simulink model "SOFC_5kW"  (Simulink 6.2)
settings: Solver=ode23tb  StartTime=0.0  StopTime=15800  MaxStep=1  RelTol=1e-3
libraries: simulink x1
settings Model: LastModifiedBy=cwang
settings DataIOCC: SaveFinalState=on  SaveOutput=off  SaveTime=off  SignalLoggingName=sigsOut
settings HardwareCC: TargetUnknown=on

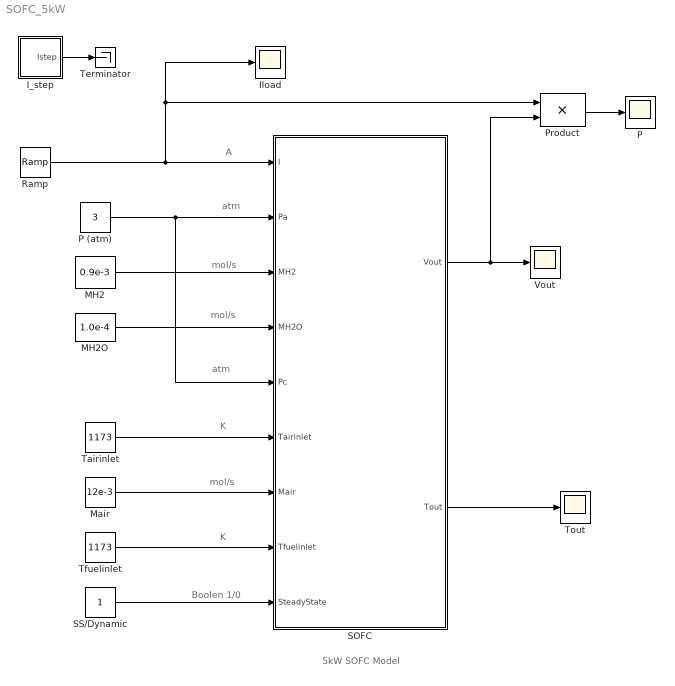
== system SOFC_5kW ==
  note: atm
  note: mol/s
  note: atm
  note: A
  note: mol/s
  note: mol/s
  note: K
  note: K
  note: 5kW SOFC Model
  note: Boolen 1/0
  I_step : Subsystem
  Iload : Scope
      settings: YMin=95  YMax=105  SaveName=Iload  DataFormat=Array
  MH2 : Constant  Value=0.9e-3
  MH2O : Constant  Value=1.0e-4
  Mair : Constant  Value=12e-3
  P : Scope
      settings: TimeRange=16000  YMin=0  YMax=5000  SaveName=Psofc  DataFormat=Array
  P (atm) : Constant  Value=3
  Product : Product  SaturateOnIntegerOverflow=on
  Ramp : simulink/Sources/Ramp  slope=0.01  start=0  X0=0
  SOFC : Subsystem
  SS/Dynamic : Constant
  Tairinlet : Constant  Value=1173
  Terminator : Terminator
  Tfuelinlet : Constant  Value=1173
  Tout : Scope
      settings: SaveName=Tout  DataFormat=Array
  Vout : Scope
      settings: SaveName=Vout  DataFormat=Array
  wires:
  P (atm)/1 -> SOFC/5(Pc), SOFC/2(Pa)
  MH2/1 -> SOFC/3(MH2)
  MH2O/1 -> SOFC/4(MH2O)
  SOFC/1(Vout) -> Vout/1, Product/2
  SOFC/2(Tout) -> Tout/1
  Tairinlet/1 -> SOFC/6(Tairinlet)
  Mair/1 -> SOFC/7(Mair)
  Tfuelinlet/1 -> SOFC/8(Tfuelinlet)
  Product/1 -> P/1
  Ramp/1 -> Iload/1, Product/1, SOFC/1(I)
  SS/Dynamic/1 -> SOFC/9(SteadyState)
  I_step/1(Istep) -> Terminator/1

== system SOFC_5kW/I_step ==
  Step : Step  Time=1000  After=80  SampleTime=0
  Step1 : Step  Time=8000  After=-50  SampleTime=0
  Sum2 : Sum  Inputs=++|  SaturateOnIntegerOverflow=on
  Istep : Outport
  wires:
  Step/1 -> Sum2/2
  Step1/1 -> Sum2/1
  Sum2/1 -> Istep/1

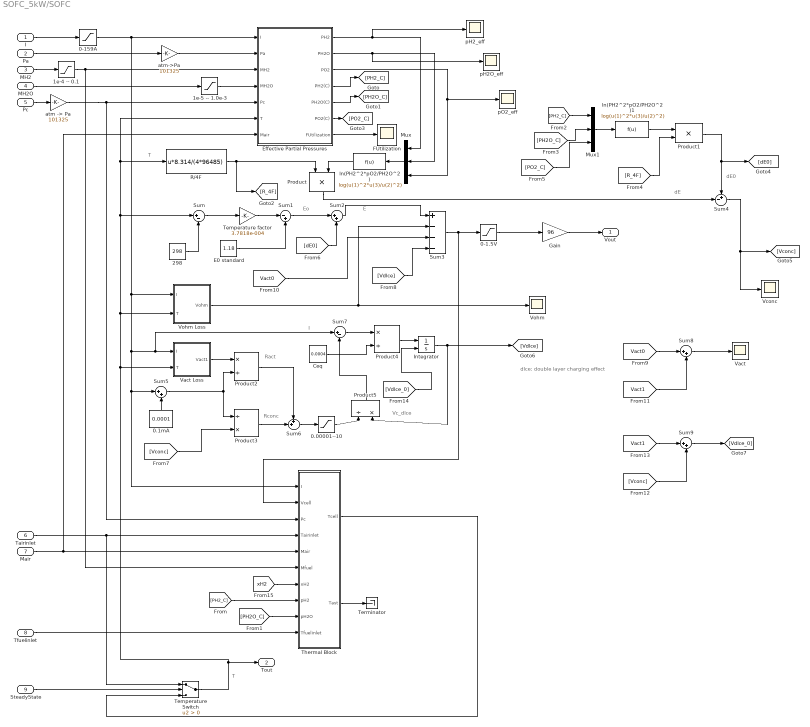
== system SOFC_5kW/SOFC ==
  note: Eo
  note: E
  note: T
  note: T
  note: dE0
  note: dE
  note: Ract
  note: Rconc
  note: I
  note: Vc_dlce
  note: dlce: double layer charging effect
  I : Inport  Port=1  LatchInput=off
  Pa : Inport  Port=2  LatchInput=off
  MH2 : Inport  Port=3  LatchInput=off
  MH2O : Inport  Port=4  LatchInput=off
  Pc : Inport  Port=5  LatchInput=off
  Tairinlet : Inport  Port=6  LatchInput=off
  Mair : Inport  Port=7  LatchInput=off
  Tfuelinlet : Inport  Port=8  LatchInput=off
  SteadyState : Inport  Port=9  LatchInput=off
  0-1.5V : Saturate  UpperLimit=1.5  LowerLimit=0
  0-159A : Saturate  UpperLimit=199  LowerLimit=0
  0.00001--10 : Saturate  UpperLimit=10  LowerLimit=0.00001
  0.1mA : Constant  Orientation=up  Value=0.0001
  "1e-4 -- 0.1" : Saturate  UpperLimit=0.1  LowerLimit=1.0e-4
  "1e-5 -- 1.0e-3" : Saturate  UpperLimit=1.0e-3  LowerLimit=1.0e-5
  298 : Constant  Value=298
  Ceq : Constant  Value=0.0004
  E0 standard : Constant  Value=1.18
  Effective Partial Pressures : Subsystem
  FUtilization : Scope
      settings: SaveName=FUtilization
  Gain : Gain  Gain=96  SaturateOnIntegerOverflow=on
  Integrator : Integrator  InitialConditionSource=external
  Mux : Mux  Orientation=left  Inputs=3
  Mux1 : Mux  Inputs=3
  Product : Product  Orientation=down  SaturateOnIntegerOverflow=on
  Product1 : Product  SaturateOnIntegerOverflow=on
  Product2 : Product  Inputs=*/  SaturateOnIntegerOverflow=on
  Product3 : Product  Inputs=/*  SaturateOnIntegerOverflow=on
  Product4 : Product  Inputs=*/  SaturateOnIntegerOverflow=on
  Product5 : Product  Orientation=up  Inputs=/*  SaturateOnIntegerOverflow=on
  R/4F : Fcn  Expr=u*8.314/(4*96485)
  Sum : Sum  Inputs=|+-  SaturateOnIntegerOverflow=on
  Sum1 : Sum  Inputs=|-+  SaturateOnIntegerOverflow=on
  Sum{2,5,8..9} (4 alike) : Sum  Inputs=|++  SaturateOnIntegerOverflow=on
  Sum3 : Sum  Inputs=+---  SaturateOnIntegerOverflow=on
  Sum4 : Sum  Inputs=+-|  SaturateOnIntegerOverflow=on
  Sum6 : Sum  Inputs=++|  SaturateOnIntegerOverflow=on
  Sum7 : Sum  Inputs=|+-  SaturateOnIntegerOverflow=on
  Temperature Switch : Switch  Criteria=u2 > Threshold  SaturateOnIntegerOverflow=on
  Temperature factor : Gain  Gain=3.7818e-004  SaturateOnIntegerOverflow=on
  Terminator : Terminator
  Thermal Block : Subsystem
  Vact : Scope
      settings: YMin=0  YMax=0.6  SaveName=Vact  DataFormat=Array
  Vact Loss : Subsystem
  Vconc : Scope
      settings: YMin=0  YMax=0.6  SaveName=Vconc  DataFormat=Array
  Vohm : Scope
      settings: YMin=0  YMax=0.6  SaveName=Vohm  DataFormat=Array
  Vohm Loss : Subsystem
  "atm -> Pa" : Gain  Gain=101325  SaturateOnIntegerOverflow=on
  atm->Pa : Gain  Gain=101325  SaturateOnIntegerOverflow=on
  ln(PH2^2*pO2/PH2O^2) : Fcn  Orientation=left  Expr=log(u(1)^2*u(3)/u(2)^2)
  ln(PH2^2*pO2/PH2O^2)1 : Fcn  Expr=log(u(1)^2*u(3)/u(2)^2)
  pH2O_eff : Scope
      settings: SaveName=pH2O_eff
  pH2_eff : Scope
      settings: TimeRange=9.779411764705881  YMin=75033  YMax=75199.9  SaveName=pH2_eff  DataFormat=Array  MaxDataPoints=10000
  pO2_eff : Scope
      settings: SaveName=pO2_eff
  Vout : Outport
  Tout : Outport  Port=2
  wires:
  Effective Partial Pressures/1(PH2) -> Mux/1, pH2_eff/1
  Pa/1 -> atm->Pa/1
  MH2/1 -> "1e-4 -- 0.1"/1
  MH2O/1 -> "1e-5 -- 1.0e-3"/1
  Effective Partial Pressures/2(PH2O) -> Mux/2, pH2O_eff/1
  Pc/1 -> "atm -> Pa"/1
  Effective Partial Pressures/3(PO2) -> pO2_eff/1, Mux/3
  298/1 -> Sum/2
  Sum/1 -> Temperature factor/1
  Temperature factor/1 -> Sum1/1
  E0 standard/1 -> Sum1/2
  Mux/1 -> ln(PH2^2*pO2/PH2O^2)/1
  R/4F/1 -> Product/1, [R_4F]
  ln(PH2^2*pO2/PH2O^2)/1 -> Product/2
  Product/1 -> Sum4/2
  I/1 -> 0-159A/1
  Sum2/1 -> Sum3/1
  Vohm Loss/1(Vohm) -> Sum3/2, Vohm/1
  Sum3/1 -> Thermal Block/2(Vcell), 0-1.5V/1
  Thermal Block/2(Tast) -> Terminator/1
  Thermal Block/1(Tcell) -> Temperature Switch/3
  atm->Pa/1 -> Effective Partial Pressures/2(Pa)
  Tairinlet/1 -> Thermal Block/4(Tairinlet), Temperature Switch/1
  Mair/1 -> Thermal Block/5(Mair), Effective Partial Pressures/7(Mair)
  "atm -> Pa"/1 -> Thermal Block/3(Pc), Effective Partial Pressures/5(Pc)
  Tfuelinlet/1 -> Thermal Block/10(Tfuelinlet)
  Effective Partial Pressures/4(PH2(C)) -> [PH2_C]
  Effective Partial Pressures/5(PH2O(C)) -> [PH2O_C]
  [PH2_C] -> Thermal Block/8(pH2)
  [PH2O_C] -> Thermal Block/9(pH2O)
  0-159A/1 -> Thermal Block/1(I), Sum5/1, Vact Loss/1(I), Sum7/1, Vohm Loss/1(I), Effective Partial Pressures/1(I)
  0-1.5V/1 -> Gain/1
  SteadyState/1 -> Temperature Switch/2
  Temperature Switch/1 -> Vohm Loss/2(T), Sum/1, Effective Partial Pressures/6(T), R/4F/1, Vact Loss/2(T), Tout/1
  Effective Partial Pressures/6(PO2(C)) -> [PO2_C]
  [PH2_C] -> Mux1/1
  [PH2O_C] -> Mux1/2
  Mux1/1 -> ln(PH2^2*pO2/PH2O^2)1/1
  ln(PH2^2*pO2/PH2O^2)1/1 -> Product1/1
  [R_4F] -> Product1/2
  Product1/1 -> Sum4/1, [dE0]
  Sum4/1 -> [Vconc], Vconc/1
  [PO2_C] -> Mux1/3
  "1e-5 -- 1.0e-3"/1 -> Effective Partial Pressures/4(MH2O)
  Effective Partial Pressures/7(FUtilization) -> FUtilization/1
  Sum1/1 -> Sum2/1
  [dE0] -> Sum2/2
  Vact Loss/1(Vact1) -> Product2/1
  0.1mA/1 -> Sum5/2
  Sum5/1 -> Product2/2, Product3/1
  Product2/1 -> Sum6/1
  [Vconc] -> Product3/2
  Sum7/1 -> Product4/1
  Ceq/1 -> Product4/2
  Product4/1 -> Integrator/1
  [Vdlce_0] -> Integrator/2
  Product3/1 -> Sum6/2
  Sum6/1 -> 0.00001--10/1
  0.00001--10/1 -> Product5/1
  Integrator/1 -> Product5/2, [Vdlce]
  Product5/1 -> Sum7/2
  [Vact0] -> Sum3/3
  [Vdlce] -> Sum3/4
  [Vact0] -> Sum8/1
  [Vact1] -> Sum8/2
  Sum8/1 -> Vact/1
  [Vact1] -> Sum9/1
  [Vconc] -> Sum9/2
  Sum9/1 -> [Vdlce_0]
  "1e-4 -- 0.1"/1 -> Effective Partial Pressures/3(MH2), Thermal Block/6(Mfuel)
  [xH2] -> Thermal Block/7(xH2)
  Gain/1 -> Vout/1

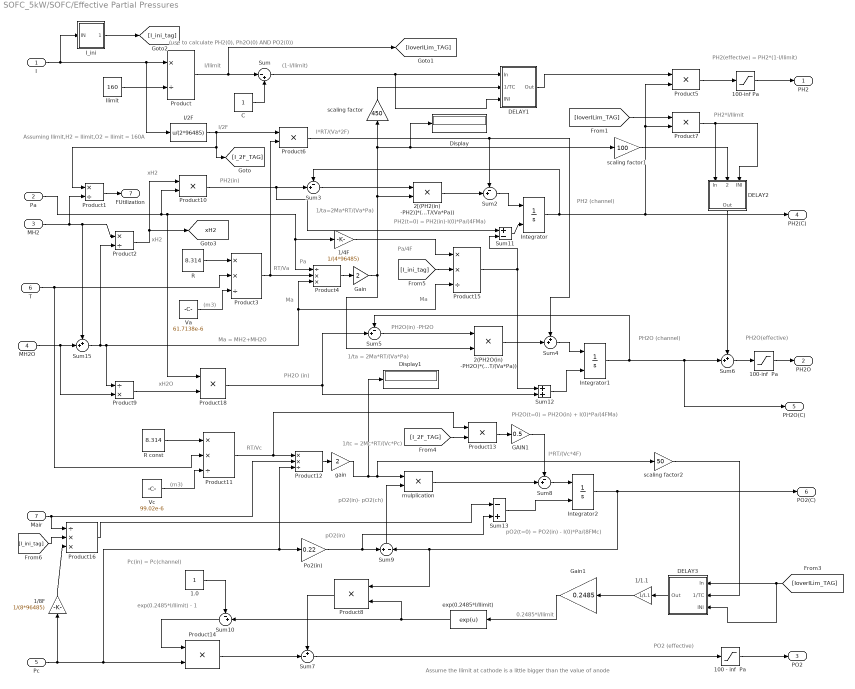
== system SOFC_5kW/SOFC/Effective Partial Pressures ==
  note: RT/Va
  note: PH2(in)
  note: 1/ta = 2Ma*RT/(Va*Pa)
  note: Pa
  note: Ma
  note: PH2(t=0) = PH2(in)-I(0)*Pa/(4FMa)
  note: I/2F
  note: I*RT/(Va*2F)
  note: PH2 (channel)
  note: PH2O(in) -PH2O
  note: PH2O(t=0) = PH2O(in) + I(0)*Pa/(4FMa)
  note: PH2O (channel)
  note: (1-I/Ilimit)
  note: Assuming Ilimit,H2 = Ilimit,O2
      |       = Ilimit = 160A
  note: I/Ilimit
  note: PH2*I/Ilimit
  note: PH2(effective) = PH2*(1-I/Ilimit)
  note: PH2O(effective)
  note: Ma = MH2+MH2O
  note: Pc(in) = Pc(channel)
  note: Assume the Ilimit at cathode is a little bigger than the value of anode
  note: 0.2485*I/Ilimit
  note: PO2 (effective)
  note: (m3)
  note: RT/Vc
  note: (m3)
  note: pO2(in)- pO2(ch)
  note: 1/tc = 2Mc*RT/(Vc*Pc)
  note: I*RT/(Vc*4F)
  note: exp(0.2485*I/Ilimit) - 1
  note: (use to calculate PH2(0), Ph2O(0) AND PO2(0))
  note: Pa/4F
  note: Ma
  note: PH2O (in)
  note: pO2(in)
  note: pO2(t=0) = PO2(in) - I(0)*Pa/(8FMc)
  note: 1/ta=2Ma*RT/(Va*Pa)
  note: xH2
  note: xH2
  note: xH2O
  I : Inport  Port=1  LatchInput=off
  Pa : Inport  Port=2  LatchInput=off
  MH2 : Inport  Port=3  LatchInput=off
  MH2O : Inport  Port=4  LatchInput=off
  Pc : Inport  Port=5  LatchInput=off
  T : Inport  Port=6  LatchInput=off
  Mair : Inport  Port=7  LatchInput=off
  1.0 : Constant
  1/1.1 : Gain  Orientation=left  Gain=1/1.1  SaturateOnIntegerOverflow=on
  1/4F : Gain  Gain=1/(4*96485)  SaturateOnIntegerOverflow=on
  1/8F : Gain  Orientation=up  Gain=1/(8*96485)  SaturateOnIntegerOverflow=on
  100 - inf  Pa : Saturate  UpperLimit=inf  LowerLimit=100
  100-inf  Pa : Saturate  UpperLimit=inf  LowerLimit=100
  100-inf Pa : Saturate  UpperLimit=inf  LowerLimit=100
  2(PH2O(in) -PH2O)*(Ma*RT/(Va*Pa)) : Product  SaturateOnIntegerOverflow=on
  2[(PH2(in) -PH2)]*(Ma*RT/(Va*Pa)) : Product  SaturateOnIntegerOverflow=on
  C : Constant
  DELAY1 : Subsystem
  DELAY2 : Subsystem  Orientation=down
  DELAY3 : Subsystem  Orientation=left
  Display : Display
  Display1 : Display
  GAIN1 : Gain  Gain=0.5  SaturateOnIntegerOverflow=on
  Gain : Gain  Gain=2  SaturateOnIntegerOverflow=on
  Gain1 : Gain  Orientation=left  Gain=0.2485  SaturateOnIntegerOverflow=on
  I/2F : Fcn  Expr=u/(2*96485)
  I_ini : Subsystem
  Ilimit : Constant  Value=160
  Integrator : Integrator  InitialConditionSource=external
  Integrator1 : Integrator  InitialConditionSource=external
  Integrator2 : Integrator  InitialConditionSource=external
  Po2(in) : Gain  Gain=0.22  SaturateOnIntegerOverflow=on
  Product : Product  Inputs=*/  SaturateOnIntegerOverflow=on
  Product1 : Product  Inputs=*/  SaturateOnIntegerOverflow=on
  Product{5..7,10,13..14,18} (7 alike) : Product  SaturateOnIntegerOverflow=on
  Product{3,11..12,15} (4 alike) : Product  Inputs=**/  SaturateOnIntegerOverflow=on
  Product16 : Product  Inputs=/**  SaturateOnIntegerOverflow=on
  Product2 : Product  Inputs=*/  SaturateOnIntegerOverflow=on
  Product4 : Product  Inputs=/**  SaturateOnIntegerOverflow=on
  Product8 : Product  Orientation=left  SaturateOnIntegerOverflow=on
  Product9 : Product  Inputs=/*  SaturateOnIntegerOverflow=on
  R : Constant  Value=8.314
  R const : Constant  Value=8.314
  Sum : Sum  Inputs=|-+  SaturateOnIntegerOverflow=on
  Sum10 : Sum  Orientation=left  Inputs=-+|  SaturateOnIntegerOverflow=on
  Sum11 : Sum  Inputs=+-  SaturateOnIntegerOverflow=on
  Sum12 : Sum  SaturateOnIntegerOverflow=on
  Sum13 : Sum  Inputs=-+  SaturateOnIntegerOverflow=on
  Sum15 : Sum  Inputs=++|  SaturateOnIntegerOverflow=on
  Sum{2..3,5,8} (4 alike) : Sum  Inputs=-+|  SaturateOnIntegerOverflow=on
  Sum4 : Sum  Inputs=++|  SaturateOnIntegerOverflow=on
  Sum6 : Sum  Inputs=++|  SaturateOnIntegerOverflow=on
  Sum7 : Sum  Inputs=+-|  SaturateOnIntegerOverflow=on
  Sum9 : Sum  Orientation=up  Inputs=+|-  SaturateOnIntegerOverflow=on
  Va : Constant  Value=61.7138e-6
  Vc : Constant  Value=99.02e-6
  exp(0.2485*I/Ilimit) : Fcn  Orientation=left  Expr=exp(u)
  gain : Gain  Gain=2  SaturateOnIntegerOverflow=on
  mulplication : Product  SaturateOnIntegerOverflow=on
  scaling factor : Gain  Orientation=up  Gain=450  SaturateOnIntegerOverflow=on
  scaling factor1 : Gain  Gain=100  SaturateOnIntegerOverflow=on
  scaling factor2 : Gain  Gain=50  SaturateOnIntegerOverflow=on
  PH2 : Outport
  PH2O : Outport  Port=2
  PO2 : Outport  Port=3
  PH2(C) : Outport  Port=4
  PH2O(C) : Outport  Port=5
  PO2(C) : Outport  Port=6
  FUtilization : Outport  Port=7
  tag scope: xH2=global
  wires:
  I/1 -> Product/1, I/2F/1, I_ini/1(IN)
  Ilimit/1 -> Product/2
  Product/1 -> Sum/1, [IoverILim_TAG]
  C/1 -> Sum/2
  R/1 -> Product3/1
  T/1 -> Product3/2, Product11/2
  Va/1 -> Product3/3
  Product4/1 -> Gain/1
  Product3/1 -> Product4/2, Product6/2
  Product10/1 -> Sum11/1, Sum3/2
  Sum3/1 -> 2[(PH2(in) -PH2)]*(Ma*RT/(Va*Pa))/1
  2[(PH2(in) -PH2)]*(Ma*RT/(Va*Pa))/1 -> Sum2/2
  I/2F/1 -> Product6/1, [I_2F_TAG], Product1/1
  Product6/1 -> Sum2/1, Sum4/1
  Integrator/1 -> Sum3/1, Product5/2, Product7/2, PH2(C)/1
  Sum2/1 -> Integrator/1
  Product18/1 -> Sum5/2, Sum12/2
  Sum5/1 -> 2(PH2O(in) -PH2O)*(Ma*RT/(Va*Pa))/1
  2(PH2O(in) -PH2O)*(Ma*RT/(Va*Pa))/1 -> Sum4/2
  Integrator1/1 -> Sum5/1, Sum6/2, PH2O(C)/1
  Sum4/1 -> Integrator1/1
  Product5/1 -> 100-inf Pa/1
  Sum6/1 -> 100-inf  Pa/1
  Pc/1 -> Product14/2, Product12/3, Po2(in)/1, 1/8F/1
  Gain1/1 -> exp(0.2485*I/Ilimit)/1
  Sum7/1 -> 100 - inf  Pa/1
  100-inf Pa/1 -> PH2/1
  100-inf  Pa/1 -> PH2O/1
  100 - inf  Pa/1 -> PO2/1
  [IoverILim_TAG] -> Product7/1
  R const/1 -> Product11/1
  Vc/1 -> Product11/3
  Product11/1 -> Product12/1, Product13/1
  Mair/1 -> Product12/2, Product16/1
  Product12/1 -> gain/1
  gain/1 -> mulplication/1, scaling factor2/1, Display1/1
  Integrator2/1 -> PO2(C)/1, Sum9/2, Product8/1
  Po2(in)/1 -> Sum9/1, Sum13/2
  Sum9/1 -> mulplication/2
  mulplication/1 -> Sum8/2
  [I_2F_TAG] -> Product13/2
  Product13/1 -> GAIN1/1
  GAIN1/1 -> Sum8/1
  Sum8/1 -> Integrator2/1
  exp(0.2485*I/Ilimit)/1 -> Sum10/2, Product8/2
  Sum10/1 -> Product14/1
  1.0/1 -> Sum10/1
  Product14/1 -> Sum7/2
  Product8/1 -> Sum7/1
  I_ini/1(IN(0)) -> [I_ini_tag]
  Sum11/1 -> Integrator/2
  1/4F/1 -> Product15/1
  [I_ini_tag] -> Product15/2
  Product15/1 -> Sum11/2, Sum12/1
  Sum12/1 -> Integrator1/2
  [I_ini_tag] -> Product16/2
  1/8F/1 -> Product16/3
  Product16/1 -> Sum13/1
  Sum13/1 -> Integrator2/2
  1/1.1/1 -> Gain1/1
  Gain/1 -> 2(PH2O(in) -PH2O)*(Ma*RT/(Va*Pa))/2, 2[(PH2(in) -PH2)]*(Ma*RT/(Va*Pa))/2, scaling factor/1, scaling factor1/1, Display/1
  Sum/1 -> DELAY1/1(In), DELAY1/3(INI)
  DELAY1/1(Out) -> Product5/1
  Product7/1 -> DELAY2/1(In), DELAY2/3(INI)
  DELAY2/1(Out) -> Sum6/1
  [IoverILim_TAG] -> DELAY3/1(In), DELAY3/3(INI)
  DELAY3/1(Out) -> 1/1.1/1
  scaling factor/1 -> DELAY1/2(1/TC)
  scaling factor1/1 -> DELAY2/2(1/TC)
  scaling factor2/1 -> DELAY3/2(1/TC)
  Sum15/1 -> Product2/2, Product4/3, Product15/3, Product9/1
  MH2O/1 -> Sum15/2, Product9/2
  MH2/1 -> Sum15/1, Product2/1, Product1/2
  Product2/1 -> Product10/1, [xH2]
  Pa/1 -> Product10/2, Product4/1, 1/4F/1, Product18/1
  Product9/1 -> Product18/2
  Product1/1 -> FUtilization/1

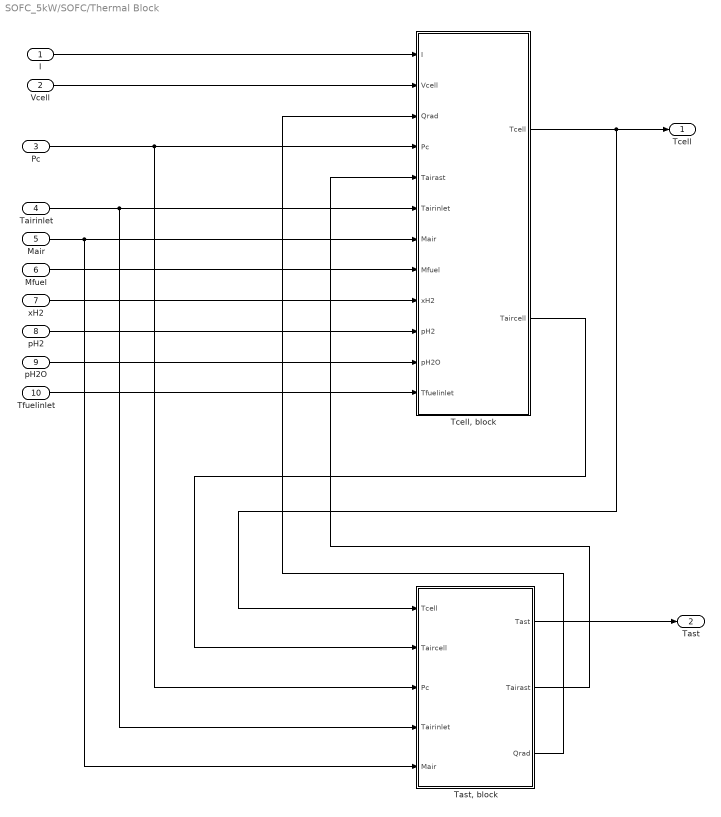
== system SOFC_5kW/SOFC/Thermal Block ==
  I : Inport  Port=1  LatchInput=off
  Vcell : Inport  Port=2  LatchInput=off
  Pc : Inport  Port=3  LatchInput=off
  Tairinlet : Inport  Port=4  LatchInput=off
  Mair : Inport  Port=5  LatchInput=off
  Mfuel : Inport  Port=6  LatchInput=off
  xH2 : Inport  Port=7  LatchInput=off
  pH2 : Inport  Port=8  LatchInput=off
  pH2O : Inport  Port=9  LatchInput=off
  Tfuelinlet : Inport  Port=10  LatchInput=off
  "Tast, block" : Subsystem
  "Tcell, block" : Subsystem
  Tcell : Outport
  Tast : Outport  Port=2
  wires:
  "Tast, block"/1(Tast) -> Tast/1
  I/1 -> "Tcell, block"/1(I)
  Vcell/1 -> "Tcell, block"/2(Vcell)
  "Tast, block"/2(Tairast) -> "Tcell, block"/5(Tairast)
  "Tast, block"/3(Qrad) -> "Tcell, block"/3(Qrad)
  "Tcell, block"/1(Tcell) -> "Tast, block"/1(Tcell), Tcell/1
  "Tcell, block"/2(Taircell) -> "Tast, block"/2(Taircell)
  Pc/1 -> "Tcell, block"/4(Pc), "Tast, block"/3(Pc)
  Tairinlet/1 -> "Tcell, block"/6(Tairinlet), "Tast, block"/4(Tairinlet)
  Mair/1 -> "Tcell, block"/7(Mair), "Tast, block"/5(Mair)
  Mfuel/1 -> "Tcell, block"/8(Mfuel)
  xH2/1 -> "Tcell, block"/9(xH2)
  pH2/1 -> "Tcell, block"/10(pH2)
  pH2O/1 -> "Tcell, block"/11(pH2O)
  Tfuelinlet/1 -> "Tcell, block"/12(Tfuelinlet)

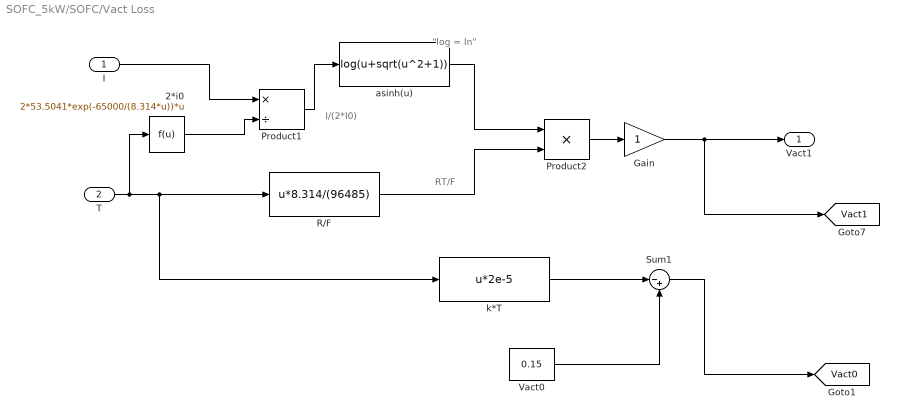
== system SOFC_5kW/SOFC/Vact Loss ==
  note: RT/F
  note: "log = ln"
  note: I/(2*I0)
  I : Inport  Port=1  LatchInput=off
  T : Inport  Port=2  LatchInput=off
  2*i0 : Fcn  Expr=2*53.5041*exp(-65000/(8.314*u))*u
  Gain : Gain  SaturateOnIntegerOverflow=on
  Product1 : Product  Inputs=*/  SaturateOnIntegerOverflow=on
  Product2 : Product  SaturateOnIntegerOverflow=on
  R/F : Fcn  Expr=u*8.314/(96485)
  Sum1 : Sum  Inputs=|-+  SaturateOnIntegerOverflow=on
  Vact0 : Constant  Value=0.15
  asinh(u) : Fcn  Expr=log(u+sqrt(u^2+1))
  k*T : Fcn  Expr=u*2e-5
  Vact1 : Outport
  tag scope: Vact0=global, Vact1=global
  wires:
  T/1 -> k*T/1, R/F/1, 2*i0/1
  R/F/1 -> Product2/2
  I/1 -> Product1/1
  Product2/1 -> Gain/1
  asinh(u)/1 -> Product2/1
  Product1/1 -> asinh(u)/1
  Gain/1 -> Vact1/1, [Vact1]
  k*T/1 -> Sum1/1
  Vact0/1 -> Sum1/2
  Sum1/1 -> [Vact0]
  2*i0/1 -> Product1/2

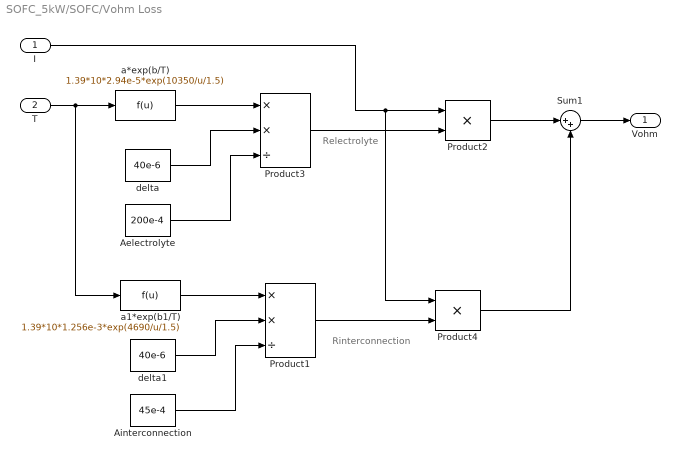
== system SOFC_5kW/SOFC/Vohm Loss ==
  note: Relectrolyte
  note: Rinterconnection
  I : Inport  Port=1  LatchInput=off
  T : Inport  Port=2  LatchInput=off
  Aelectrolyte : Constant  Value=200e-4
  Ainterconnection : Constant  Value=45e-4
  Product1 : Product  Inputs=**/  SaturateOnIntegerOverflow=on
  Product2 : Product  SaturateOnIntegerOverflow=on
  Product3 : Product  Inputs=**/  SaturateOnIntegerOverflow=on
  Product4 : Product  SaturateOnIntegerOverflow=on
  Sum1 : Sum  Inputs=|++  SaturateOnIntegerOverflow=on
  a*exp(b/T) : Fcn  Expr=1.39*10*2.94e-5*exp(10350/u/1.5)
  a1*exp(b1/T) : Fcn  Expr=1.39*10*1.256e-3*exp(4690/u/1.5)
  delta : Constant  Value=40e-6
  delta1 : Constant  Value=40e-6
  Vohm : Outport
  wires:
  T/1 -> a1*exp(b1/T)/1, a*exp(b/T)/1
  a*exp(b/T)/1 -> Product3/1
  delta/1 -> Product3/2
  Aelectrolyte/1 -> Product3/3
  Product3/1 -> Product2/2
  a1*exp(b1/T)/1 -> Product1/1
  delta1/1 -> Product1/2
  Ainterconnection/1 -> Product1/3
  Product1/1 -> Product4/2
  I/1 -> Product4/1, Product2/1
  Product2/1 -> Sum1/1
  Product4/1 -> Sum1/2
  Sum1/1 -> Vohm/1

== system SOFC_5kW/SOFC/Effective Partial Pressures/DELAY1 ==
  note: time constant
  In : Inport  Port=1  LatchInput=off
  1/TC : Inport  Port=2  LatchInput=off
  INI : Inport  Port=3  LatchInput=off
  Integrator : Integrator  InitialConditionSource=external
  Product1 : Product  SaturateOnIntegerOverflow=on
  Sum : Sum  Inputs=|+-  SaturateOnIntegerOverflow=on
  Out : Outport
  wires:
  Sum/1 -> Product1/2
  Integrator/1 -> Sum/2, Out/1
  Product1/1 -> Integrator/1
  1/TC/1 -> Product1/1
  In/1 -> Sum/1
  INI/1 -> Integrator/2

== system SOFC_5kW/SOFC/Effective Partial Pressures/DELAY2 ==
  note: time constant
  In : Inport  Port=1  LatchInput=off
  1/TC : Inport  Port=2  LatchInput=off
  INI : Inport  Port=3  LatchInput=off
  Integrator : Integrator  InitialConditionSource=external
  Product1 : Product  SaturateOnIntegerOverflow=on
  Sum : Sum  Inputs=|+-  SaturateOnIntegerOverflow=on
  Out : Outport
  wires:
  Sum/1 -> Product1/2
  Integrator/1 -> Sum/2, Out/1
  Product1/1 -> Integrator/1
  1/TC/1 -> Product1/1
  In/1 -> Sum/1
  INI/1 -> Integrator/2

== system SOFC_5kW/SOFC/Effective Partial Pressures/DELAY3 ==
  note: time constant
  In : Inport  Port=1  LatchInput=off
  1/TC : Inport  Port=2  LatchInput=off
  INI : Inport  Port=3  LatchInput=off
  Integrator : Integrator  InitialConditionSource=external
  Product1 : Product  SaturateOnIntegerOverflow=on
  Sum : Sum  Inputs=|+-  SaturateOnIntegerOverflow=on
  Out : Outport
  wires:
  Sum/1 -> Product1/2
  Integrator/1 -> Sum/2, Out/1
  Product1/1 -> Integrator/1
  1/TC/1 -> Product1/1
  In/1 -> Sum/1
  INI/1 -> Integrator/2

== system SOFC_5kW/SOFC/Effective Partial Pressures/I_ini ==
  IN : Inport  Port=1  LatchInput=off
  Integrator : Integrator  InitialConditionSource=external
  zero : Constant  Value=0
  IN(0) : Outport
  wires:
  zero/1 -> Integrator/1
  Integrator/1 -> IN(0)/1
  IN/1 -> Integrator/2

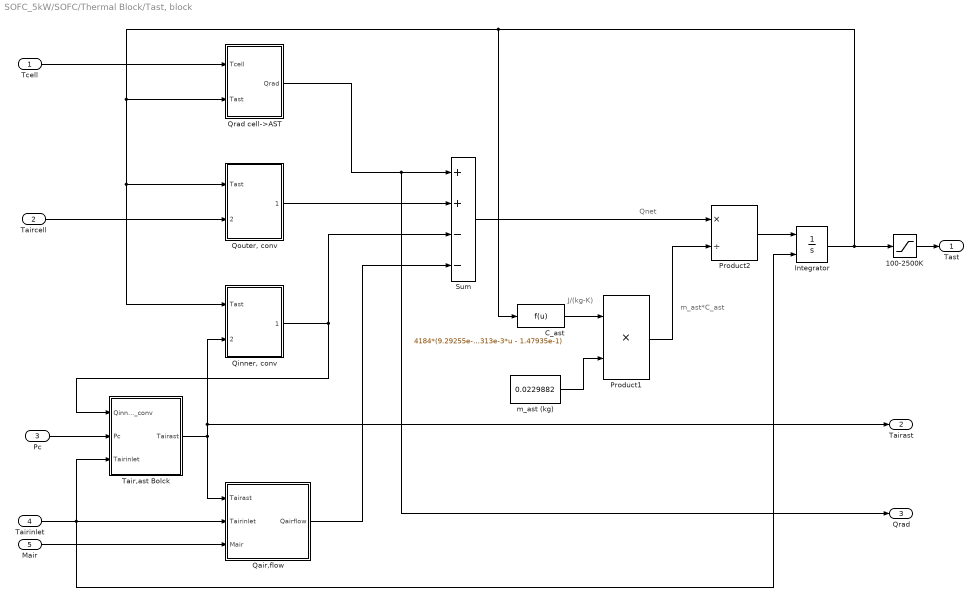
== system SOFC_5kW/SOFC/Thermal Block/Tast, block ==
  note: Qnet
  note: m_ast*C_ast
  note: J/(kg-K)
  Tcell : Inport  Port=1  LatchInput=off
  Taircell : Inport  Port=2  LatchInput=off
  Pc : Inport  Port=3  LatchInput=off
  Tairinlet : Inport  Port=4  LatchInput=off
  Mair : Inport  Port=5  LatchInput=off
  100-2500K : Saturate  UpperLimit=2500  LowerLimit=100
  C_ast : Fcn  Expr=4184*(9.29255e-20*u^6 + 6.58097e-17*u^5 - 1.55425e-12*u^4 + 3.66895e-9*u^3 - 3.79619e-6*u^2 + 1.96313e-3*u - 1.47935e-1)
  Integrator : Integrator  InitialConditionSource=external
  Product1 : Product  SaturateOnIntegerOverflow=on
  Product2 : Product  Inputs=*/  SaturateOnIntegerOverflow=on
  Qair,flow : Subsystem
  "Qinner, conv" : Subsystem
  "Qouter, conv" : Subsystem
  Qrad cell->AST : Subsystem
  Sum : Sum  Inputs=++--  SaturateOnIntegerOverflow=on
  Tair,ast Bolck : Subsystem
  m_ast (kg) : Constant  Value=0.0229882
  Tast : Outport
  Tairast : Outport  Port=2
  Qrad : Outport  Port=3
  wires:
  Tcell/1 -> Qrad cell->AST/1(Tcell)
  Qrad cell->AST/1(Qrad) -> Qrad/1, Sum/1
  Taircell/1 -> "Qouter, conv"/2(Taircell)
  Tairinlet/1 -> Integrator/2, Tair,ast Bolck/3(Tairinlet), Qair,flow/2(Tairinlet)
  Mair/1 -> Qair,flow/3(Mair)
  "Qinner, conv"/1(Qinner-conv) -> Tair,ast Bolck/1(Qinner_conv), Sum/3
  Tair,ast Bolck/1(Tairast) -> "Qinner, conv"/2(Tairast), Tairast/1, Qair,flow/1(Tairast)
  "Qouter, conv"/1(Qouter-conv) -> Sum/2
  Qair,flow/1(Qairflow) -> Sum/4
  Sum/1 -> Product2/1
  Integrator/1 -> Qrad cell->AST/2(Tast), "Qouter, conv"/1(Tast), "Qinner, conv"/1(Tast), C_ast/1, 100-2500K/1
  C_ast/1 -> Product1/1
  m_ast (kg)/1 -> Product1/2
  Product1/1 -> Product2/2
  Product2/1 -> Integrator/1
  Pc/1 -> Tair,ast Bolck/2(Pc)
  100-2500K/1 -> Tast/1

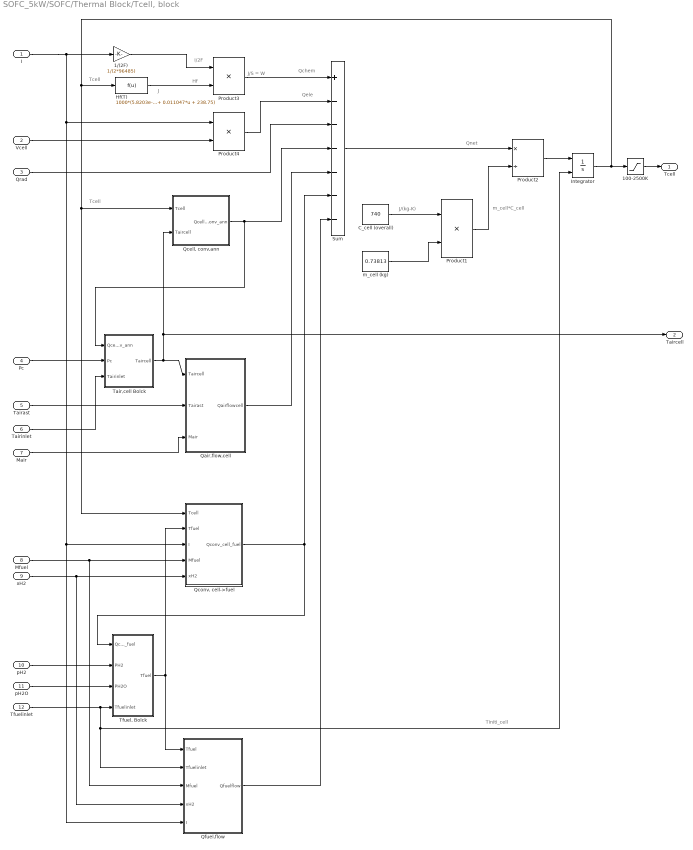
== system SOFC_5kW/SOFC/Thermal Block/Tcell, block ==
  note: Qnet
  note: m_cell*C_cell
  note: J/(kg-K)
  note: J
  note: Hf
  note: i/2F
  note: J/S = W
  note: Qchem
  note: Qele
  note: Tcell
  note: Tcell
  note: Tiniti_cell
  I : Inport  Port=1  LatchInput=off
  Vcell : Inport  Port=2  LatchInput=off
  Qrad : Inport  Port=3  LatchInput=off
  Pc : Inport  Port=4  LatchInput=off
  Tairast : Inport  Port=5  LatchInput=off
  Tairinlet : Inport  Port=6  LatchInput=off
  Mair : Inport  Port=7  LatchInput=off
  Mfuel : Inport  Port=8  LatchInput=off
  xH2 : Inport  Port=9  LatchInput=off
  pH2 : Inport  Port=10  LatchInput=off
  pH2O : Inport  Port=11  LatchInput=off
  Tfuelinlet : Inport  Port=12  LatchInput=off
  1/(2F) : Gain  Gain=1/(2*96485)  SaturateOnIntegerOverflow=on
  100-2500K : Saturate  UpperLimit=2500  LowerLimit=100
  "C_cell (overall) " : Constant  Value=740
  Hf(T) : Fcn  Expr=1000*(5.8203e-013*u^4 - 2.2337e-009*u^3 - 1.0957e-007*u^2 + 0.011047*u + 238.75)
  Integrator : Integrator  InitialConditionSource=external
  Product1 : Product  SaturateOnIntegerOverflow=on
  Product2 : Product  Inputs=*/  SaturateOnIntegerOverflow=on
  Product3 : Product  SaturateOnIntegerOverflow=on
  Product4 : Product  SaturateOnIntegerOverflow=on
  Qair,flow,cell : Subsystem
  "Qcell, conv,ann" : Subsystem
  "Qconv, cell->fuel" : Subsystem
  Qfuel,flow : Subsystem
  Sum : Sum  Inputs=+------  SaturateOnIntegerOverflow=on
  Tair,cell Bolck : Subsystem
  "Tfuel, Bolck" : Subsystem
  m_cell (kg) : Constant  Value=0.73813
  Tcell : Outport
  Taircell : Outport  Port=2
  wires:
  Tairinlet/1 -> Tair,cell Bolck/3(Tairinlet)
  Mair/1 -> Qair,flow,cell/3(Mair)
  Sum/1 -> Product2/1
  Integrator/1 -> "Qconv, cell->fuel"/1(Tcell), "Qcell, conv,ann"/1(Tcell), Hf(T)/1, 100-2500K/1
  "C_cell (overall) "/1 -> Product1/1
  m_cell (kg)/1 -> Product1/2
  Product1/1 -> Product2/2
  Product2/1 -> Integrator/1
  Pc/1 -> Tair,cell Bolck/2(Pc)
  Hf(T)/1 -> Product3/2
  I/1 -> 1/(2F)/1, Product4/1, "Qconv, cell->fuel"/3(I), Qfuel,flow/5(I)
  1/(2F)/1 -> Product3/1
  Product3/1 -> Sum/1
  Vcell/1 -> Product4/2
  Product4/1 -> Sum/2
  Qrad/1 -> Sum/3
  "Qcell, conv,ann"/1(Qcell_conv_ann) -> Tair,cell Bolck/1(Qcell_conv_ann), Sum/4
  Qair,flow,cell/1(Qairflowcell) -> Sum/5
  Tair,cell Bolck/1(Taircell) -> Qair,flow,cell/1(Taircell), "Qcell, conv,ann"/2(Taircell), Taircell/1
  Tairast/1 -> Qair,flow,cell/2(Tairast)
  "Qconv, cell->fuel"/1(Qconv_cell_fuel) -> "Tfuel, Bolck"/1(Qconv_cell_fuel), Sum/6
  "Tfuel, Bolck"/1(Tfuel) -> "Qconv, cell->fuel"/2(Tfuel), Qfuel,flow/1(Tfuel)
  Mfuel/1 -> "Qconv, cell->fuel"/4(Mfuel), Qfuel,flow/3(Mfuel)
  xH2/1 -> "Qconv, cell->fuel"/5(xH2), Qfuel,flow/4(xH2)
  pH2/1 -> "Tfuel, Bolck"/2(PH2)
  pH2O/1 -> "Tfuel, Bolck"/3(PH2O)
  Tfuelinlet/1 -> "Tfuel, Bolck"/4(Tfuelinlet), Qfuel,flow/2(Tfuelinlet), Integrator/2
  Qfuel,flow/1(Qfuelflow) -> Sum/7
  100-2500K/1 -> Tcell/1

== system SOFC_5kW/SOFC/Thermal Block/Tast, block/Qair,flow ==
  note: Tair,exit, AST- Tair,inlet,AST = 2*(Tair,AST- Tair,inlet,AST)
  note: mol/s
  note: J/(Kg-K)
  note: Kg/s
  Tairast : Inport  Port=1  LatchInput=off
  Tairinlet : Inport  Port=2  LatchInput=off
  Mair : Inport  Port=3  LatchInput=off
  Cair : Fcn  Expr=1.9327e-10*u^4 - 7.9999e-7*u^3 + 1.1407e-3*u^2 - 4.489e-1*u + 1.0575e3
  Gain : Gain  Gain=2  SaturateOnIntegerOverflow=on
  Product2 : Product  Inputs=3  SaturateOnIntegerOverflow=on
  Sum2 : Sum  Inputs=|+-  SaturateOnIntegerOverflow=on
  molecular weight of air : Gain  Gain=28.95*1e-3  SaturateOnIntegerOverflow=on
  Qairflow : Outport
  wires:
  Product2/1 -> Qairflow/1
  Tairast/1 -> Sum2/1, Cair/1
  Tairinlet/1 -> Sum2/2
  Mair/1 -> molecular weight of air/1
  Sum2/1 -> Gain/1
  Gain/1 -> Product2/1
  Cair/1 -> Product2/3
  molecular weight of air/1 -> Product2/2

== system SOFC_5kW/SOFC/Thermal Block/Tast, block/Qinner, conv ==
  note: hast,2
  Tast : Inport  Port=1  LatchInput=off
  Tairast : Inport  Port=2  LatchInput=off
  Aast (m2) : Constant  Value=62.2035e-4
  Dast : Constant  Value=0.396e-2
  Kfair : Fcn  Expr=1.5207e-11*u^3 - 4.8574e-8*u^2 + 1.0184e-4*u - 3.9333e-4
  Product1 : Product  Inputs=**/  SaturateOnIntegerOverflow=on
  Product2 : Product  Inputs=3  SaturateOnIntegerOverflow=on
  Sum2 : Sum  Inputs=|+-  SaturateOnIntegerOverflow=on
  effective Nusselt number : Constant  Value=4.364
  Qinner-conv : Outport
  wires:
  Product2/1 -> Qinner-conv/1
  Tast/1 -> Sum2/1, Kfair/1
  Tairast/1 -> Sum2/2
  Aast (m2)/1 -> Product2/2
  Sum2/1 -> Product2/1
  effective Nusselt number/1 -> Product1/1
  Kfair/1 -> Product1/2
  Dast/1 -> Product1/3
  Product1/1 -> Product2/3

== system SOFC_5kW/SOFC/Thermal Block/Tast, block/Qouter, conv ==
  note: hast,1
  Tast : Inport  Port=1  LatchInput=off
  Taircell : Inport  Port=2  LatchInput=off
  Aast (m2) : Constant  Value=87.022e-4
  Dh,ast : Constant  Value=0.626e-2
  Kfair : Fcn  Expr=1.5207e-11*u^3 - 4.8574e-8*u^2 + 1.0184e-4*u - 3.9333e-4
  Product1 : Product  Inputs=**/  SaturateOnIntegerOverflow=on
  Product2 : Product  Inputs=3  SaturateOnIntegerOverflow=on
  Sum2 : Sum  Inputs=|-+  SaturateOnIntegerOverflow=on
  effective Nusselt number : Constant  Value=4.076
  Qouter-conv : Outport
  wires:
  Product2/1 -> Qouter-conv/1
  Tast/1 -> Sum2/1, Kfair/1
  Taircell/1 -> Sum2/2
  Aast (m2)/1 -> Product2/2
  Sum2/1 -> Product2/1
  effective Nusselt number/1 -> Product1/1
  Kfair/1 -> Product1/2
  Dh,ast/1 -> Product1/3
  Product1/1 -> Product2/3

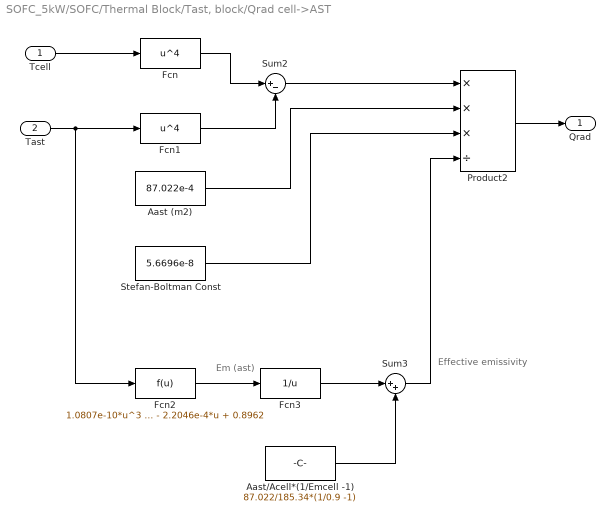
== system SOFC_5kW/SOFC/Thermal Block/Tast, block/Qrad cell->AST ==
  note: Effective emissivity
  note: Em (ast)
  Tcell : Inport  Port=1  LatchInput=off
  Tast : Inport  Port=2  LatchInput=off
  Aast (m2) : Constant  Value=87.022e-4
  Aast/Acell*(1/Emcell -1) : Constant  Value=87.022/185.34*(1/0.9 -1)
  Fcn : Fcn  Expr=u^4
  Fcn1 : Fcn  Expr=u^4
  Fcn2 : Fcn  Expr=1.0807e-10*u^3 - 2.4164e-7*u^2 - 2.2046e-4*u + 0.8962
  Fcn3 : Fcn  Expr=1/u
  Product2 : Product  Inputs=***/  SaturateOnIntegerOverflow=on
  Stefan-Boltman Const : Constant  Value=5.6696e-8
  Sum2 : Sum  Inputs=|+-  SaturateOnIntegerOverflow=on
  Sum3 : Sum  Inputs=|++  SaturateOnIntegerOverflow=on
  Qrad : Outport
  wires:
  Product2/1 -> Qrad/1
  Tcell/1 -> Fcn/1
  Tast/1 -> Fcn1/1, Fcn2/1
  Sum3/1 -> Product2/4
  Aast/Acell*(1/Emcell -1)/1 -> Sum3/2
  Fcn3/1 -> Sum3/1
  Fcn2/1 -> Fcn3/1
  Stefan-Boltman Const/1 -> Product2/3
  Aast (m2)/1 -> Product2/2
  Sum2/1 -> Product2/1
  Fcn1/1 -> Sum2/2
  Fcn/1 -> Sum2/1

== system SOFC_5kW/SOFC/Thermal Block/Tast, block/Tair,ast Bolck ==
  note: J/(Kg-K)
  note: mol/s
  note: mair*Cpair =
      | Heat Capacity
  note: Kg/s
  note: Tair,ast
  note: Unit = N/(m2)
  note: Vast*Pc/(RT)
  Qinner_conv : Inport  Port=1  LatchInput=off
  Pc : Inport  Port=2  LatchInput=off
  Tairinlet : Inport  Port=3  LatchInput=off
  100-2500K : Saturate  UpperLimit=2500  LowerLimit=100
  Cpair : Fcn  Expr=1.9327e-10*u^4 - 7.9999e-7*u^3 + 1.1407e-3*u^2 - 4.489e-1*u + 1.0575e3
  Integrator : Integrator  InitialConditionSource=external
  Product1 : Product  SaturateOnIntegerOverflow=on
  Product2 : Product  Inputs=*/  SaturateOnIntegerOverflow=on
  Product3 : Product  Inputs=**/  SaturateOnIntegerOverflow=on
  RT : Gain  Orientation=left  Gain=8.314  SaturateOnIntegerOverflow=on
  Vast,cave (m3) : Constant  Value=6.1581e-6
  molecular weight of air : Gain  Gain=28.95*1e-3  SaturateOnIntegerOverflow=on
  Tairast : Outport
  wires:
  Qinner_conv/1 -> Product2/1
  Product1/1 -> Product2/2
  Product2/1 -> Integrator/1
  Integrator/1 -> Cpair/1, RT/1, 100-2500K/1
  Tairinlet/1 -> Integrator/2
  Pc/1 -> Product3/1
  Cpair/1 -> Product1/1
  Vast,cave (m3)/1 -> Product3/2
  Product3/1 -> molecular weight of air/1
  RT/1 -> Product3/3
  molecular weight of air/1 -> Product1/2
  100-2500K/1 -> Tairast/1

== system SOFC_5kW/SOFC/Thermal Block/Tcell, block/Qair,flow,cell ==
  note: Tair,exit, CELL- Tair,exit,AST ~ (Tair,CELL- Tair, AST)
  note: mol/s
  note: J/(Kg-K)
  note: Kg/s
  Taircell : Inport  Port=1  LatchInput=off
  Tairast : Inport  Port=2  LatchInput=off
  Mair : Inport  Port=3  LatchInput=off
  Cair : Fcn  Expr=1.9327e-10*u^4 - 7.9999e-7*u^3 + 1.1407e-3*u^2 - 4.489e-1*u + 1.0575e3
  Gain : Gain  SaturateOnIntegerOverflow=on
  Product2 : Product  Inputs=3  SaturateOnIntegerOverflow=on
  Sum1 : Sum  Inputs=+-  SaturateOnIntegerOverflow=on
  molecular weight of air : Gain  Gain=28.95*1e-3  SaturateOnIntegerOverflow=on
  Qairflowcell : Outport
  wires:
  Product2/1 -> Qairflowcell/1
  Tairast/1 -> Sum1/2
  Mair/1 -> molecular weight of air/1
  Gain/1 -> Product2/1
  Cair/1 -> Product2/3
  molecular weight of air/1 -> Product2/2
  Taircell/1 -> Sum1/1, Cair/1
  Sum1/1 -> Gain/1

== system SOFC_5kW/SOFC/Thermal Block/Tcell, block/Qcell, conv,ann ==
  note: hcell
  Tcell : Inport  Port=1  LatchInput=off
  Taircell : Inport  Port=2  LatchInput=off
  Acell (m2) : Constant  Value=185.34e-4
  Dh : Constant  Value=0.626e-2
  Kfair : Fcn  Expr=1.5207e-11*u^3 - 4.8574e-8*u^2 + 1.0184e-4*u - 3.9333e-4
  Product1 : Product  Inputs=**/  SaturateOnIntegerOverflow=on
  Product2 : Product  Inputs=3  SaturateOnIntegerOverflow=on
  Sum2 : Sum  Inputs=|+-  SaturateOnIntegerOverflow=on
  effective Nusselt number : Constant  Value=4.169/(1+0.2042)
  Qcell_conv_ann : Outport
  wires:
  Product2/1 -> Qcell_conv_ann/1
  Tcell/1 -> Kfair/1, Sum2/1
  Taircell/1 -> Sum2/2
  Acell (m2)/1 -> Product2/2
  Sum2/1 -> Product2/1
  effective Nusselt number/1 -> Product1/1
  Kfair/1 -> Product1/2
  Dh/1 -> Product1/3
  Product1/1 -> Product2/3

== system SOFC_5kW/SOFC/Thermal Block/Tcell, block/Qconv, cell->fuel ==
  note: hcf
  note: kfuel
  note: W/(m-K)
  Tcell : Inport  Port=1  LatchInput=off
  Tfuel : Inport  Port=2  LatchInput=off
  I : Inport  Port=3  LatchInput=off
  Mfuel : Inport  Port=4  LatchInput=off
  xH2 : Inport  Port=5  LatchInput=off
  Acell (m2) : Constant  Value=185.34e-4
  Dh : Constant  Value=0.644e-2
  Product1 : Product  Inputs=**/  SaturateOnIntegerOverflow=on
  Product2 : Product  Inputs=3  SaturateOnIntegerOverflow=on
  Sum2 : Sum  Inputs=|+-  SaturateOnIntegerOverflow=on
  effective Nusselt number : Constant  Value=5.9
  kfuel,block : Subsystem
  Qconv_cell_fuel : Outport
  wires:
  Product2/1 -> Qconv_cell_fuel/1
  Tcell/1 -> Sum2/1
  Tfuel/1 -> Sum2/2, kfuel,block/1(Tfuel)
  Acell (m2)/1 -> Product2/2
  Sum2/1 -> Product2/1
  Dh/1 -> Product1/3
  Product1/1 -> Product2/3
  effective Nusselt number/1 -> Product1/2
  I/1 -> kfuel,block/2(I)
  xH2/1 -> kfuel,block/4(xH2)
  Mfuel/1 -> kfuel,block/3(Mfuel)
  kfuel,block/1(kfuel) -> Product1/1

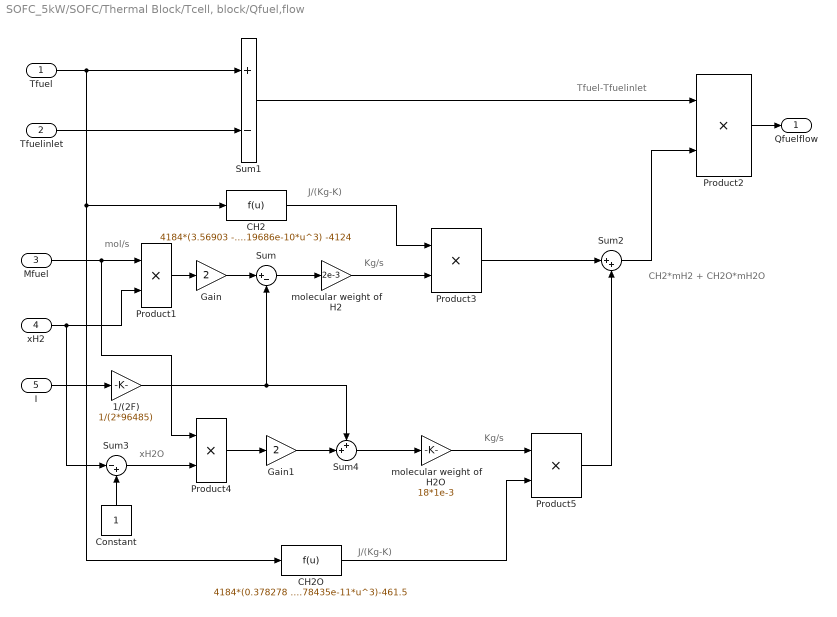
== system SOFC_5kW/SOFC/Thermal Block/Tcell, block/Qfuel,flow ==
  note: mol/s
  note: J/(Kg-K)
  note: Kg/s
  note: Tfuel-Tfuelinlet
  note: J/(Kg-K)
  note: Kg/s
  note: xH2O
  note: CH2*mH2 + CH2O*mH2O
  Tfuel : Inport  Port=1  LatchInput=off
  Tfuelinlet : Inport  Port=2  LatchInput=off
  Mfuel : Inport  Port=3  LatchInput=off
  xH2 : Inport  Port=4  LatchInput=off
  I : Inport  Port=5  LatchInput=off
  1/(2F) : Gain  Gain=1/(2*96485)  SaturateOnIntegerOverflow=on
  CH2 : Fcn  Expr=4184*(3.56903 -4.8950e-4*u + 6.22549e-7*u^2 - 1.19686e-10*u^3) -4124
  CH2O : Fcn  Expr=4184*(0.378278 + 1.53443e-4*u + 3.31531e-8*u^2 - 1.78435e-11*u^3)-461.5
  Constant : Constant  Orientation=up
  Gain : Gain  Gain=2  SaturateOnIntegerOverflow=on
  Gain1 : Gain  Gain=2  SaturateOnIntegerOverflow=on
  Product{1..5} (5 alike) : Product  SaturateOnIntegerOverflow=on
  Sum : Sum  Inputs=|+-  SaturateOnIntegerOverflow=on
  Sum1 : Sum  Inputs=+-  SaturateOnIntegerOverflow=on
  Sum2 : Sum  Inputs=|++  SaturateOnIntegerOverflow=on
  Sum3 : Sum  Inputs=|-+  SaturateOnIntegerOverflow=on
  Sum4 : Sum  Inputs=++|  SaturateOnIntegerOverflow=on
  molecular weight of H2 : Gain  Gain=2e-3  SaturateOnIntegerOverflow=on
  molecular weight of H2O : Gain  Gain=18*1e-3  SaturateOnIntegerOverflow=on
  Qfuelflow : Outport
  wires:
  Product2/1 -> Qfuelflow/1
  Tfuel/1 -> Sum1/1, CH2/1, CH2O/1
  Tfuelinlet/1 -> Sum1/2
  Sum1/1 -> Product2/1
  Mfuel/1 -> Product1/1, Product4/1
  xH2/1 -> Product1/2, Sum3/1
  I/1 -> 1/(2F)/1
  1/(2F)/1 -> Sum/2, Sum4/1
  Product1/1 -> Gain/1
  Sum/1 -> molecular weight of H2/1
  molecular weight of H2/1 -> Product3/2
  Sum2/1 -> Product2/2
  CH2/1 -> Product3/1
  Gain/1 -> Sum/1
  Constant/1 -> Sum3/2
  Sum3/1 -> Product4/2
  Product4/1 -> Gain1/1
  Gain1/1 -> Sum4/2
  Sum4/1 -> molecular weight of H2O/1
  Product3/1 -> Sum2/1
  molecular weight of H2O/1 -> Product5/1
  CH2O/1 -> Product5/2
  Product5/1 -> Sum2/2

== system SOFC_5kW/SOFC/Thermal Block/Tcell, block/Tair,cell Bolck ==
  note: J/(Kg-K)
  note: mol/s
  note: mair*Cpair =
      | Heat Capacity
  note: Kg/s
  note: Tair,cell
  note: Unit = N/(m2)
  note: Vann*Pc/(RT)
  Qcell_conv_ann : Inport  Port=1  LatchInput=off
  Pc : Inport  Port=2  LatchInput=off
  Tairinlet : Inport  Port=3  LatchInput=off
  100-2500K : Saturate  UpperLimit=2500  LowerLimit=100
  Cair : Fcn  Expr=1.9327e-10*u^4 - 7.9999e-7*u^3 + 1.1407e-3*u^2 - 4.489e-1*u + 1.0575e3
  Integrator : Integrator  InitialConditionSource=external
  Product1 : Product  SaturateOnIntegerOverflow=on
  Product2 : Product  Inputs=*/  SaturateOnIntegerOverflow=on
  Product3 : Product  Inputs=**/  SaturateOnIntegerOverflow=on
  RT : Gain  Orientation=left  Gain=8.314  SaturateOnIntegerOverflow=on
  Vann (m3) : Constant  Value=42.6269e-6
  molecular weight of air : Gain  Gain=28.95*1e-3  SaturateOnIntegerOverflow=on
  Taircell : Outport
  wires:
  Qcell_conv_ann/1 -> Product2/1
  Product1/1 -> Product2/2
  Product2/1 -> Integrator/1
  Integrator/1 -> Cair/1, RT/1, 100-2500K/1
  Tairinlet/1 -> Integrator/2
  Pc/1 -> Product3/1
  Cair/1 -> Product1/1
  Vann (m3)/1 -> Product3/2
  Product3/1 -> molecular weight of air/1
  RT/1 -> Product3/3
  molecular weight of air/1 -> Product1/2
  100-2500K/1 -> Taircell/1

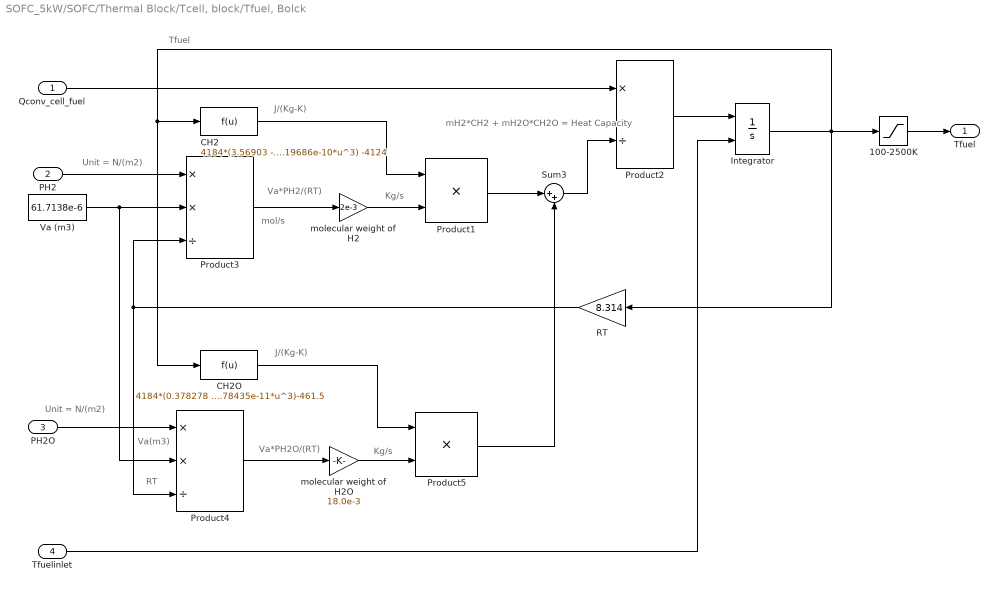
== system SOFC_5kW/SOFC/Thermal Block/Tcell, block/Tfuel, Bolck ==
  note: J/(Kg-K)
  note: mol/s
  note: mH2*CH2 + mH2O*CH2O =
      | Heat Capacity
  note: Kg/s
  note: Tfuel
  note: Unit = N/(m2)
  note: Va*PH2/(RT)
  note: Unit = N/(m2)
  note: Va(m3)
  note: RT
  note: Va*PH2O/(RT)
  note: J/(Kg-K)
  note: Kg/s
  Qconv_cell_fuel : Inport  Port=1  LatchInput=off
  PH2 : Inport  Port=2  LatchInput=off
  PH2O : Inport  Port=3  LatchInput=off
  Tfuelinlet : Inport  Port=4  LatchInput=off
  100-2500K : Saturate  UpperLimit=2500  LowerLimit=100
  CH2 : Fcn  Expr=4184*(3.56903 -4.8950e-4*u + 6.22549e-7*u^2 - 1.19686e-10*u^3) -4124
  CH2O : Fcn  Expr=4184*(0.378278 + 1.53443e-4*u + 3.31531e-8*u^2 - 1.78435e-11*u^3)-461.5
  Integrator : Integrator  InitialConditionSource=external
  Product1 : Product  SaturateOnIntegerOverflow=on
  Product2 : Product  Inputs=*/  SaturateOnIntegerOverflow=on
  Product3 : Product  Inputs=**/  SaturateOnIntegerOverflow=on
  Product4 : Product  Inputs=**/  SaturateOnIntegerOverflow=on
  Product5 : Product  SaturateOnIntegerOverflow=on
  RT : Gain  Orientation=left  Gain=8.314  SaturateOnIntegerOverflow=on
  Sum3 : Sum  Inputs=|++  SaturateOnIntegerOverflow=on
  Va (m3) : Constant  Value=61.7138e-6
  molecular weight of H2 : Gain  Gain=2e-3  SaturateOnIntegerOverflow=on
  molecular weight of H2O : Gain  Gain=18.0e-3  SaturateOnIntegerOverflow=on
  Tfuel : Outport
  wires:
  Qconv_cell_fuel/1 -> Product2/1
  Product2/1 -> Integrator/1
  Integrator/1 -> RT/1, CH2/1, CH2O/1, 100-2500K/1
  Tfuelinlet/1 -> Integrator/2
  PH2/1 -> Product3/1
  CH2/1 -> Product1/1
  Va (m3)/1 -> Product3/2, Product4/2
  Product3/1 -> molecular weight of H2/1
  RT/1 -> Product3/3, Product4/3
  molecular weight of H2/1 -> Product1/2
  PH2O/1 -> Product4/1
  Product4/1 -> molecular weight of H2O/1
  molecular weight of H2O/1 -> Product5/2
  CH2O/1 -> Product5/1
  Product1/1 -> Sum3/1
  Product5/1 -> Sum3/2
  Sum3/1 -> Product2/2
  100-2500K/1 -> Tfuel/1

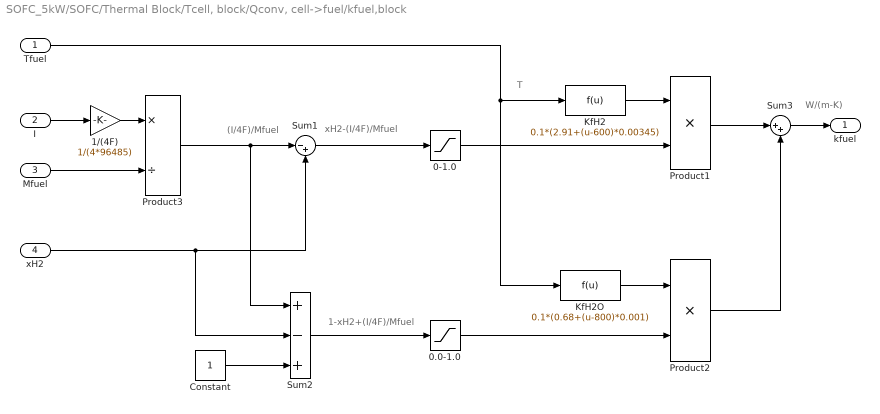
== system SOFC_5kW/SOFC/Thermal Block/Tcell, block/Qconv, cell->fuel/kfuel,block ==
  note: (I/4F)/Mfuel
  note: xH2-(I/4F)/Mfuel
  note: 1-xH2+(I/4F)/Mfuel
  note: T
  note: W/(m-K)
  Tfuel : Inport  Port=1  LatchInput=off
  I : Inport  Port=2  LatchInput=off
  Mfuel : Inport  Port=3  LatchInput=off
  xH2 : Inport  Port=4  LatchInput=off
  0-1.0 : Saturate  UpperLimit=1  LowerLimit=0
  0.0-1.0 : Saturate  UpperLimit=1  LowerLimit=0
  1/(4F) : Gain  Gain=1/(4*96485)  SaturateOnIntegerOverflow=on
  Constant : Constant
  KfH2 : Fcn  Expr=0.1*(2.91+(u-600)*0.00345)
  KfH2O : Fcn  Expr=0.1*(0.68+(u-800)*0.001)
  Product1 : Product  SaturateOnIntegerOverflow=on
  Product2 : Product  SaturateOnIntegerOverflow=on
  Product3 : Product  Inputs=*/  SaturateOnIntegerOverflow=on
  Sum1 : Sum  Inputs=|-+  SaturateOnIntegerOverflow=on
  Sum2 : Sum  Inputs=+-+  SaturateOnIntegerOverflow=on
  Sum3 : Sum  Inputs=|++  SaturateOnIntegerOverflow=on
  kfuel : Outport
  wires:
  I/1 -> 1/(4F)/1
  1/(4F)/1 -> Product3/1
  Mfuel/1 -> Product3/2
  Product3/1 -> Sum1/1, Sum2/1
  xH2/1 -> Sum2/2, Sum1/2
  Sum1/1 -> 0-1.0/1
  Constant/1 -> Sum2/3
  Sum2/1 -> 0.0-1.0/1
  Tfuel/1 -> KfH2O/1, KfH2/1
  KfH2/1 -> Product1/1
  0-1.0/1 -> Product1/2
  KfH2O/1 -> Product2/1
  0.0-1.0/1 -> Product2/2
  Product1/1 -> Sum3/1
  Product2/1 -> Sum3/2
  Sum3/1 -> kfuel/1
